simulink model "Copy_3_of_CDPR_q"  (R2023b)
settings: Solver=FixedStepAuto  StartTime=0.0  StopTime=10  FixedStep=0.001  RelTol=1e-3
values from neighbouring files (symbols this model uses):
  R = (sqrt(0.08^2 + 0.005^2/(2*pi))/25)    [DynModel_q.m]    (also in Initialisation.m = (sqrt(0.08^2 + 0.005^2/(2*pi))/25)   * eye(8); Rot.m = Rz * Ry * Rx; Rz.m = [cos(theta) -sin(theta) 0)
  tau_ci = quadprog(H, f, [], [], Aeq, beq, 50*ones(8,1), 5000*ones(8,1))    [Initialisation.m]    (also in TDA.m = u(13:20))
  Xi = [0, 0.0, 2.2, 0, 0, 0]'    [Initialisation.m]
settings Model: Creator=abellila  LastModifiedBy=abellila
settings SolverCC: SolverJacobianMethodControl=FullAnalytical

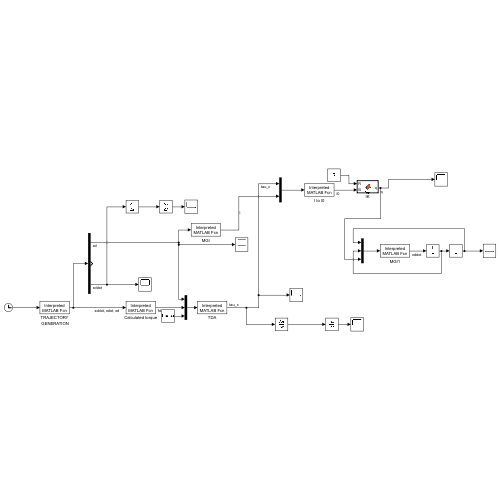
[thumbnail: Simulink's stored preview of the top-level diagram]
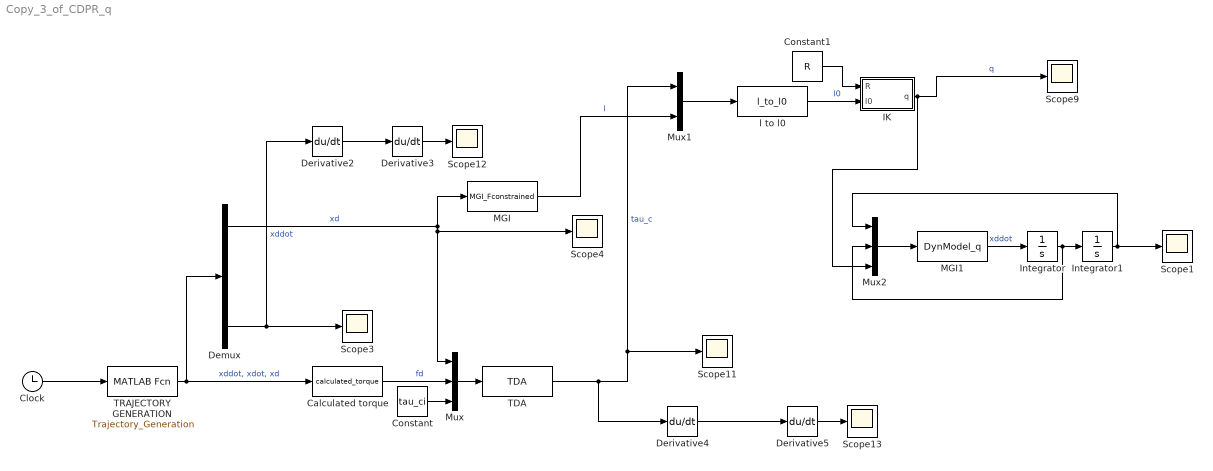
== system Copy_3_of_CDPR_q ==
  Calculated torque : MATLABFcn  MATLABFcn=calculated_torque  Output1D=off
  Clock : Clock
  Constant : Constant  Value=tau_ci
  Constant1 : Constant  Value=R
  Demux : Demux  Outputs=3
  Derivative{2..5} (4 alike) : Derivative
  IK : MATLAB Function  TreatAsAtomicUnit=on
  Integrator : Integrator
  Integrator1 : Integrator  InitialCondition=Xi
  MGI : MATLABFcn  MATLABFcn=MGI_Fconstrained
  MGI1 : MATLABFcn  MATLABFcn=DynModel_q  OutputDimensions=6  Output1D=off
  Mux : Mux  Inputs=3
  Mux1 : Mux  Inputs=2
  Mux2 : Mux  Inputs=3
  Scope{1,3..4,9,11..13} (7 alike) : Scope
  TDA : MATLABFcn  MATLABFcn=TDA  OutputDimensions=8  Output1D=off
  TRAJECTORY GENERATION : MATLABFcn  MATLABFcn=Trajectory_Generation  Output1D=off
  l to l0 : MATLABFcn  MATLABFcn=l_to_l0  OutputDimensions=8  OutputSignalType=real  Output1D=off
  wires:
  Derivative4/1 -> Derivative5/1
  Derivative5/1 -> Scope13/1
  Derivative2/1 -> Derivative3/1
  Clock/1 -> TRAJECTORY GENERATION/1
  Constant1/1 -> IK/1(R)
  Mux/1 -> TDA/1
  Demux/1 -> Mux/1, Scope4/1, MGI/1  "xd"
  IK/1(q) -> Mux2/3, Scope9/1  "q"
  TDA/1 -> Derivative4/1, Scope11/1, Mux1/1  "tau_c"
  TRAJECTORY GENERATION/1 -> Calculated torque/1, Demux/1  "xddot, xdot, xd"
  Demux/3 -> Derivative2/1, Scope3/1  "xddot"
  Constant/1 -> Mux/3
  Derivative3/1 -> Scope12/1
  MGI/1 -> Mux1/2  "l"
  Calculated torque/1 -> Mux/2  "fd"
  l to l0/1 -> IK/2(l0)  "l0"
  Mux1/1 -> l to l0/1
  Mux2/1 -> MGI1/1
  MGI1/1 -> Integrator/1  "xddot"
  Integrator/1 -> Mux2/2, Integrator1/1
  Integrator1/1 -> Mux2/1, Scope1/1

== matlab function Copy_3_of_CDPR_q/IK ==
  data: R input; q output; l0 input
function q = fcn(R, l0)

q = R\l0;
